simulink library "Valve"  (R2018b)
settings: Solver=ode45  StartTime=0.0  StopTime=10.0  RelTol=1e-3  EnableMultiTasking=on
undefined symbols (not defined in the file): DPConstant, DPLinear, DPQuadratic, ID, linear, Pressure
libraries: carnot x2
settings Model: Creator=lena.frank  LastModifiedBy=P41573
settings DataIOCC: LimitDataPoints=on  SaveFormat=Array  SignalLoggingSaveFormat=ModelDataLogs
settings OptimizationCC: ExpressionDepthLimit=2147483647  LifeSpan=inf
settings DebuggingCC: UnderspecifiedInitializationDetection=Classic  MergeDetectMultiDrivingBlocksExec=none  SolverPrmCheckMsg=warning  FcnCallInpInsideContextMsg=warning  StateNameClashWarn=warning  SFUnexpectedBacktrackingDiag=warning  SFNoUnconditionalDefaultTransitionDiag=warning  SFExecutionAtInitializationDiag=none
settings HardwareCC: ProdBitPerPointer=32  ProdBitPerSizeT=32  ProdBitPerPtrDiffT=32  ProdLargestAtomicFloat=None  ProdIntDivRoundTo=Undefined  ProdEndianess=Unspecified  ProdWordSize=32  ProdHWDeviceType=32-bit Generic
settings ModelReferenceCC: PropagateSignalLabelsOutOfModel=off
settings SFSimCC: SimUseLocalCustomCode=off
settings RTWCC: RTWUseLocalCustomCode=off
settings CodeAppCC: StateflowObjectComments=on
settings GRTTargetCC: TargetLangStandard=C89/C90 (ANSI)  GeneratePreprocessorConditionals=Disable all  CombineOutputUpdateFcns=off  GRTInterface=on
settings ConfigComp: CovMetricSettings=dw  CovHtmlReporting=on  CovSaveCumulativeToWorkspaceVar=on  CovSaveSingleToWorkspaceVar=on  CovExternalEMLEnable=off

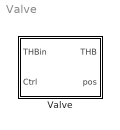
== system Valve ==
  Valve : Subsystem  mask(Valve Function){vtyp=linear, psi_0=0.04, kvs=1.6, dt_V=30}
      mask prompts: vtyp "Valve characteristic"; psi_0 "Psi_0: relative flow coefficient Kv/Kvs of the closed valve"; kvs "Kvs: flow coefficient of the open valve in m³/h"; dt_V "Valve running time in s"
      mask help:
      | Model of a valve with flow coefficient characteristic:
      | Linear                     psi = psi_0 + (1-psi_0)*h
      | Equal percentage    psi = psi_0 * (1/psi_0)^h)
      | with
      |   h = H/H100   relative opening
      |   Kv                 flow coefficient in m³/h
      |   Kv = Vdot * sqrt(1e5Pa/dp * density/1000kg/m³)
      |   Kvs                flow coefficient  in m³/h of the fully opened valve.
      |   psi = Kv/Kvs  relative flow coefficient
      |   Vdot             volumetric flow rate in m³/h
      | Typical value for the relative flow coefficient at zero opening psi_0 is 0.04
      mask Help: web(fullfile(path_carnot('help'),'Valve.html'),'-helpbrowser')
      mask TypeOptions vtyp: relFlowCoefficientFunction/vtyp
      mask TypeOptions psi_0: relFlowCoefficientFunction/psi_0
      mask TypeOptions kvs: relFlowCoeff2qua/kvs
      mask TypeOptions dt_V: Rate Limiter/dt_V
      mask Display:
      | plot(-30,-20,130,120,[10,90,90,10,10],[50,0,50,0,50],...
      |     [50,50],[50,25],...
      |     [40,30,30,40,60,70,70,60,40],[50,60,80,90,90,80,60,50,50],...
      |     [60,60,50,40,40],[60,80,70,80,60])

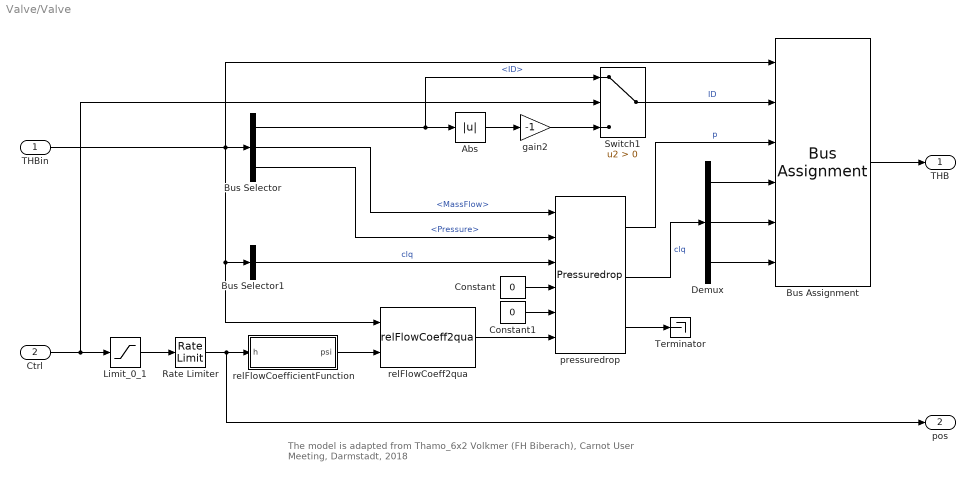
== system Valve/Valve ==
  note: The model is adapted from Thamo_6x2
      | Volkmer (FH Biberach), Carnot User Meeting, Darmstadt, 2018
  THBin : Inport
  Ctrl : Inport  Port=2
  Abs : Abs
  Bus Assignment : BusAssignment  AssignedSignals=ID,Pressure,DPConstant,DPLinear,DPQuadratic
  Bus Selector : BusSelector  OutputSignals=ID,MassFlow,Pressure
  Bus Selector1 : BusSelector  OutputSignals=DPConstant,DPLinear,DPQuadratic  OutputAsBus=on
  Constant : Constant  Value=0
  Constant1 : Constant  Value=0
  Demux : Demux  Outputs=3
  Limit_0_1 : Saturate  UpperLimit=1  LowerLimit=0
  Rate Limiter : RateLimiter  RisingSlewLimit=1/dt_V  FallingSlewLimit=-1/dt_V  SampleTimeMode=inherited  mask{dt_V=dt_V}
      mask prompts: dt_V "Valve running time in s"
  Switch1 : Switch  Criteria=u2 > Threshold  SaturateOnIntegerOverflow=on  InputSameDT=on
  Terminator : Terminator
  gain2 : Gain  Gain=-1  SaturateOnIntegerOverflow=on  OutDataTypeStr=Inherit: Same as input  ParamDataTypeStr=Inherit: Same as input
  pressuredrop : carnot/Basic/Pressure_Drop/Pressuredrop
      settings: SourceProductName=Carnot
  relFlowCoeff2qua : carnot/Basic/Pressure_Drop/relFlowCoeff2qua  kvs=kvs
      settings: SourceProductName=Carnot
  relFlowCoefficientFunction : Subsystem  mask{vtyp=linear, psi_0=psi_0}
      mask prompts: vtyp "Valve characteristic"; psi_0 "Relative flow coefficient at zero opening"
      mask TypeOptions vtyp: linear | equal percentage
      mask TypeOptions psi_0: EqualPercentageCharacteristic/psi_0 | LinearCharacteristic/psi_0 | defaultLinear/psi_0
      mask Display: disp('rel\nFlow Coeff')
  THB : Outport
  pos : Outport  Port=2
  wires:
  Demux/3 -> Bus Assignment/6
  Demux/2 -> Bus Assignment/5
  Demux/1 -> Bus Assignment/4
  Bus Assignment/1 -> THB/1
  THBin/1 -> Bus Assignment/1, Bus Selector1/1, relFlowCoeff2qua/1, Bus Selector/1
  pressuredrop/3 -> Terminator/1
  Constant1/1 -> pressuredrop/5
  Constant/1 -> pressuredrop/4
  pressuredrop/2 -> Demux/1  "clq"
  Bus Selector/3 -> pressuredrop/2  "<Pressure>"
  Abs/1 -> gain2/1
  Switch1/1 -> Bus Assignment/2  "ID"
  Bus Selector/2 -> pressuredrop/1  "<MassFlow>"
  pressuredrop/1 -> Bus Assignment/3  "p"
  Bus Selector1/1 -> pressuredrop/3  "clq"
  Ctrl/1 -> Switch1/2, Limit_0_1/1
  Bus Selector/1 -> Abs/1, Switch1/1  "<ID>"
  gain2/1 -> Switch1/3
  relFlowCoefficientFunction/1(psi) -> relFlowCoeff2qua/2
  Limit_0_1/1 -> Rate Limiter/1
  relFlowCoeff2qua/1 -> pressuredrop/6
  Rate Limiter/1 -> relFlowCoefficientFunction/1(h), pos/1

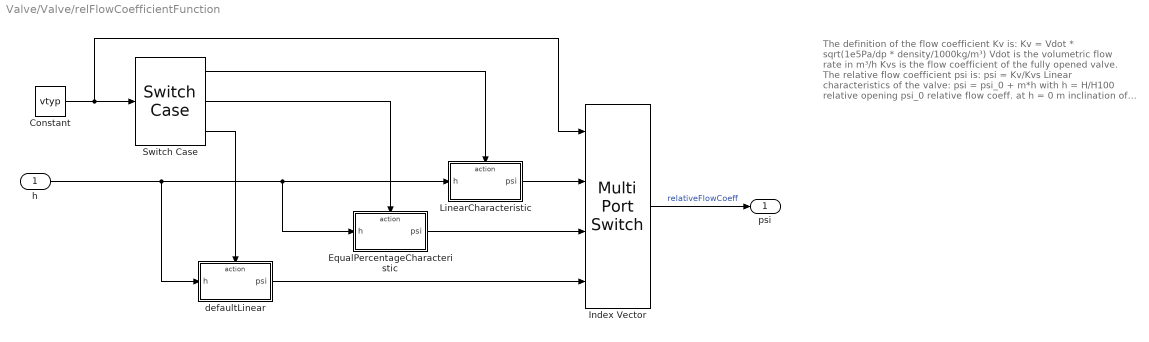
== system Valve/Valve/relFlowCoefficientFunction ==
  note: The definition of the flow coefficient Kv is:
      | Kv = Vdot * sqrt(1e5Pa/dp * density/1000kg/m³)
      | Vdot is the volumetric flow rate in m³/h
      | Kvs is the flow coefficient of the fully opened valve.
      | The relative flow coefficient psi is:
      | psi = Kv/Kvs
      |
      | Linear characteristics of the valve:
      | psi = psi_0 + m*h
      | with
      | h = H/H100 relative opening
      | psi_0 relative flow coeff. at h = 0
      | m inclination of the linear equation
      | psi should be 1 when h = 1, so: m = (1-psi_0)
      | psi = psi_0 + (1-psi_0)*h
      |
      | Equal percentage characteristics of the valve:
      | psi = psi_0 * e^(n*h)
      | with
      | n = ln(1/psi_0) inclination of the characteristics
      | the relative flow coefficient is:
      | psi = psi_0 * (1/psi_0)^h)
  h : Inport
  Constant : Constant  Value=vtyp
  EqualPercentageCharacteristic : Subsystem  TreatAsAtomicUnit=on  mask{psi_0=psi_0}
      mask prompts: psi_0 "Relative flow coefficient at zero opening"
      mask TypeOptions psi_0: psi_0/Value
  Index Vector : MultiPortSwitch
  LinearCharacteristic : Subsystem  TreatAsAtomicUnit=on  mask{psi_0=psi_0}
      mask prompts: psi_0 "Relative flow coefficient at zero opening"
      mask TypeOptions psi_0: psi_0/Value
  Switch Case : SwitchCase  CaseConditions={1,2}
  defaultLinear : Subsystem  TreatAsAtomicUnit=on  mask{psi_0=psi_0}
      mask prompts: psi_0 "Relative flow coefficient at zero opening"
      mask TypeOptions psi_0: psi_0/Value
  psi : Outport
  wires:
  Index Vector/1 -> psi/1  "relativeFlowCoeff"
  Constant/1 -> Index Vector/1, Switch Case/1
  Switch Case/1 -> LinearCharacteristic/Action
  h/1 -> defaultLinear/1(h), EqualPercentageCharacteristic/1(h), LinearCharacteristic/1(h)
  LinearCharacteristic/1(psi) -> Index Vector/2
  Switch Case/2 -> EqualPercentageCharacteristic/Action
  Switch Case/3 -> defaultLinear/Action
  EqualPercentageCharacteristic/1(psi) -> Index Vector/3
  defaultLinear/1(psi) -> Index Vector/4

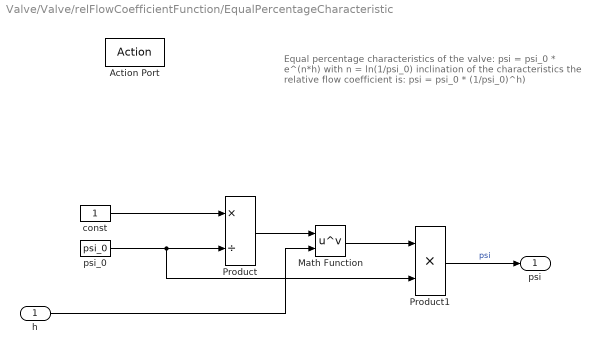
== system Valve/Valve/relFlowCoefficientFunction/EqualPercentageCharacteristic ==
  note: Equal percentage characteristics of the valve:
      | psi = psi_0 * e^(n*h)
      | with
      | n = ln(1/psi_0) inclination of the characteristics
      | the relative flow coefficient is:
      | psi = psi_0 * (1/psi_0)^h)
  h : Inport
  Action Port : ActionPort
  Math Function : Math  Operator=pow  SaturateOnIntegerOverflow=on
  Product : Product  Inputs=*/
  Product1 : Product
  const : Constant
  psi_0 : Constant  Value=psi_0
  psi : Outport
  wires:
  Product1/1 -> psi/1  "psi"
  const/1 -> Product/1
  psi_0/1 -> Product1/2, Product/2
  Product/1 -> Math Function/1
  h/1 -> Math Function/2
  Math Function/1 -> Product1/1

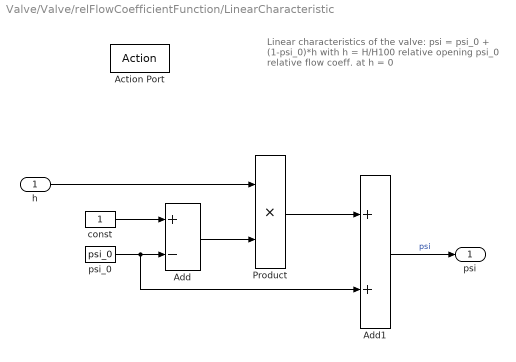
== system Valve/Valve/relFlowCoefficientFunction/LinearCharacteristic ==
  note: Linear characteristics of the valve:
      | psi = psi_0 + (1-psi_0)*h
      | with
      | h = H/H100 relative opening
      | psi_0 relative flow coeff. at h = 0
  h : Inport
  Action Port : ActionPort
  Add : Sum  Inputs=+-
  Add1 : Sum  Inputs=2
  Product : Product
  const : Constant
  psi_0 : Constant  Value=psi_0
  psi : Outport
  wires:
  const/1 -> Add/1
  psi_0/1 -> Add1/2, Add/2
  Add/1 -> Product/2
  h/1 -> Product/1
  Product/1 -> Add1/1
  Add1/1 -> psi/1  "psi"

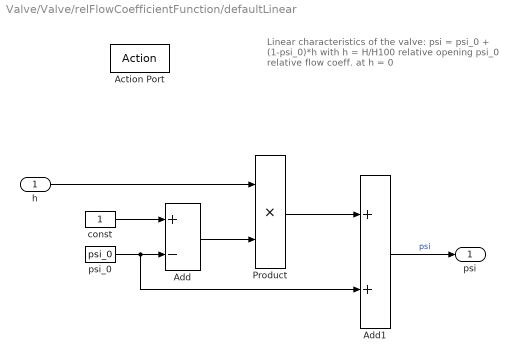
== system Valve/Valve/relFlowCoefficientFunction/defaultLinear ==
  note: Linear characteristics of the valve:
      | psi = psi_0 + (1-psi_0)*h
      | with
      | h = H/H100 relative opening
      | psi_0 relative flow coeff. at h = 0
  h : Inport
  Action Port : ActionPort
  Add : Sum  Inputs=+-
  Add1 : Sum  Inputs=2
  Product : Product
  const : Constant
  psi_0 : Constant  Value=psi_0
  psi : Outport
  wires:
  Add1/1 -> psi/1  "psi"
  Product/1 -> Add1/1
  h/1 -> Product/1
  Add/1 -> Product/2
  psi_0/1 -> Add/2, Add1/2
  const/1 -> Add/1
